simulink model "model2x2PulsedCA1ECMay1_2005"  (Simulink 7.1)
settings: Solver=ode45  StartTime=0.0  StopTime=100  RelTol=1e-3
settings Model: Creator=Terri Murray  LastModifiedBy=Terri Murray
settings DataIOCC: LimitDataPoints=off
settings OptimizationCC: InlineInvariantSignals=on
settings DebuggingCC: SaveWithParameterizedLinksMsg=none  SignalResolutionControl=TryResolveAllWithWarning  MultiTaskDSMMsg=warning  MultiTaskCondExecSysMsg=none  StrictBusMsg=None
settings RTWCC: IncludeERTFirstTime=on
settings GRTTargetCC: TargetFcnLib=ansi_tfl_tmw.mat

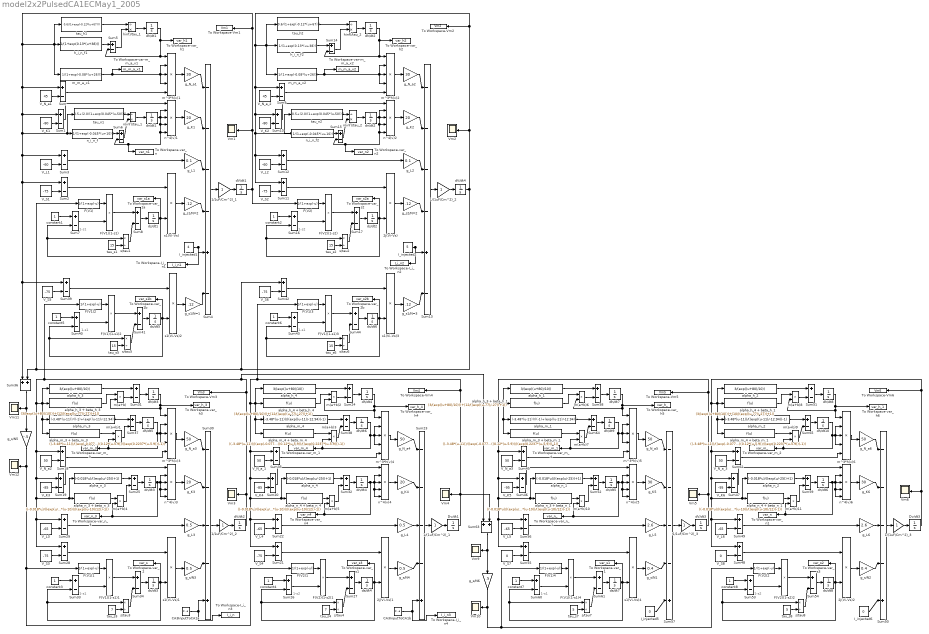
== system model2x2PulsedCA1ECMay1_2005 ==
  note: 1-s1
  note: 1-s2
  note: 1-s1
  note: 1-s2
  note: 1-s1
  note: 1-s1
  note: 1-s1
  note: 1-s2
  " 1/(1uF/Cm^2)_1" : Gain  ParameterDataType=sfix(16)  ParameterScaling=2^0  OutDataType=sfix(16)  OutScaling=2^0  SaturateOnIntegerOverflow=on  OutDataTypeStr=Inherit: Same as input  ParamDataTypeStr=Inherit: Same as input
  " 1/(1uF/Cm^2)_2" : Gain  ParameterDataType=sfix(16)  ParameterScaling=2^0  OutDataType=sfix(16)  OutScaling=2^0  SaturateOnIntegerOverflow=on  OutDataTypeStr=Inherit: Same as input  ParamDataTypeStr=Inherit: Same as input
  " 1/(1uF/Cm^2)_3" : Gain  ParameterDataType=sfix(16)  ParameterScaling=2^0  OutDataType=sfix(16)  OutScaling=2^0  SaturateOnIntegerOverflow=on  OutDataTypeStr=Inherit: Same as input  ParamDataTypeStr=Inherit: Same as input
  " 1/1uF/Cm^2)_1" : Gain  ParameterDataType=sfix(16)  ParameterScaling=2^0  OutDataType=sfix(16)  OutScaling=2^0  SaturateOnIntegerOverflow=on  OutDataTypeStr=Inherit: Same as input  ParamDataTypeStr=Inherit: Same as input
  " 1/1uF/Cm^2)_2" : Gain  ParameterDataType=sfix(16)  ParameterScaling=2^0  OutDataType=sfix(16)  OutScaling=2^0  SaturateOnIntegerOverflow=on  OutDataTypeStr=Inherit: Same as input  ParamDataTypeStr=Inherit: Same as input
  " 1/1uF/Cm^2)_3" : Gain  ParameterDataType=sfix(16)  ParameterScaling=2^0  OutDataType=sfix(16)  OutScaling=2^0  SaturateOnIntegerOverflow=on  OutDataTypeStr=Inherit: Same as input  ParamDataTypeStr=Inherit: Same as input
  2j(Vi-Vs) : Product  OutDataType=sfix(16)  OutScaling=2^0  RndMeth=Zero
  2j(Vi-Vs)1 : Product  OutDataType=sfix(16)  OutScaling=2^0  RndMeth=Zero
  2j(Vi-Vs)2 : Product  OutDataType=sfix(16)  OutScaling=2^0  RndMeth=Zero
  CA3InputToCA1a : DiscretePulseGenerator  PulseType=Time based  Amplitude=200  Period=.02  PulseWidth=2  PhaseDelay=.5
  CA3InputToCA1b : DiscretePulseGenerator  PulseType=Time based  Amplitude=200  Period=.02  PulseWidth=2
  Dv/dt1 : Integrator  InitialCondition=-67.6
  Dv/dt3 : Integrator  InitialCondition=-68
  F(V1){,1..4} (5 alike) : Fcn  Expr=1/(1+exp(-u))
  F(V1)(1-s1){,1..4} (5 alike) : Product  OutDataType=sfix(16)  OutScaling=2^0  RndMeth=Zero
  F(V2) : Fcn  Expr=1/(1+exp(-u))
  F(V2)(1-s2) : Product  OutDataType=sfix(16)  OutScaling=2^0  RndMeth=Zero
  F(V2)(1-s2)1 : Product  OutDataType=sfix(16)  OutScaling=2^0  RndMeth=Zero
  F(V2)(1-s2)2 : Product  OutDataType=sfix(16)  OutScaling=2^0  RndMeth=Zero
  F(V2)1 : Fcn  Expr=1/(1+exp(-u))
  F(V2)2 : Fcn  Expr=1/(1+exp(-u))
  I_injected1 : Constant  Value=4  OutDataType=sfix(16)  OutScaling=2^0
  I_injected2 : Constant  Value=5  OutDataType=sfix(16)  OutScaling=2^0
  I_injected5 : Constant  Value=0  OutDataType=sfix(16)  OutScaling=2^0
  I_injected6 : Constant  Value=0  OutDataType=sfix(16)  OutScaling=2^0
  Sum{,1..3,5..12,14..22,24..29,31..35,37..49,51..56,58..62,64..65} (58 alike) : Sum  Inputs=+-  OutDataType=sfix(16)  OutScaling=2^0  SaturateOnIntegerOverflow=on
  Sum13 : Sum  Inputs=-||-||-||-||+|||-  OutDataType=sfix(16)  OutScaling=2^0  SaturateOnIntegerOverflow=on
  Sum{23,30,50,57} (4 alike) : Sum  Inputs=-||-||-||-||+  OutDataType=sfix(16)  OutScaling=2^0  SaturateOnIntegerOverflow=on
  Sum36 : Sum  Orientation=down  OutDataType=sfix(16)  OutScaling=2^0  SaturateOnIntegerOverflow=on
  Sum4 : Sum  Inputs=-||-||-||-||+|||-  OutDataType=sfix(16)  OutScaling=2^0  SaturateOnIntegerOverflow=on
  Sum63 : Sum  Orientation=down  OutDataType=sfix(16)  OutScaling=2^0  SaturateOnIntegerOverflow=on
  To Workspace-I_i_n1 : ToWorkspace  VariableName=I_i_n1  SampleTime=-1  SaveFormat=Array
  To Workspace-I_i_n2 : ToWorkspace  VariableName=I_i_n2  SampleTime=-1  SaveFormat=Array
  To Workspace-I_i_n3 : ToWorkspace  VariableName=I_i_n  SampleTime=-1  SaveFormat=Array
  To Workspace-I_i_n4 : ToWorkspace  VariableName=I_i_n3  SampleTime=-1  SaveFormat=Array
  To Workspace-Vm1 : ToWorkspace  VariableName=Vm1  SampleTime=-1  SaveFormat=Array
  To Workspace-Vm2 : ToWorkspace  VariableName=Vm2  SampleTime=-1  SaveFormat=Array
  To Workspace-Vm3 : ToWorkspace  VariableName=Vm3  SampleTime=-1  SaveFormat=Array
  To Workspace-Vm4 : ToWorkspace  VariableName=Vm4  SampleTime=-1  SaveFormat=Array
  To Workspace-Vm5 : ToWorkspace  VariableName=Vm5  SampleTime=-1  SaveFormat=Array
  To Workspace-Vm6 : ToWorkspace  VariableName=Vm6  SampleTime=-1  SaveFormat=Array
  To Workspace-var-m_m_a_x1 : ToWorkspace  VariableName=m_m_a_x1  SampleTime=-1  SaveFormat=Array
  To Workspace-var-m_m_a_x2 : ToWorkspace  VariableName=m_m_a_x2  SampleTime=-1  SaveFormat=Array
  To Workspace-var_1 : ToWorkspace  VariableName=var_s1  SampleTime=-1  SaveFormat=Array
  To Workspace-var_1a : ToWorkspace  VariableName=var_s1a  SampleTime=-1  SaveFormat=Array
  To Workspace-var_1b : ToWorkspace  VariableName=var_s1b  SampleTime=-1  SaveFormat=Array
  To Workspace-var_2 : ToWorkspace  VariableName=var_s  SampleTime=-1  SaveFormat=Array
  To Workspace-var_2b : ToWorkspace  VariableName=var_s2b  SampleTime=-1  SaveFormat=Array
  To Workspace-var_h1 : ToWorkspace  VariableName=var_h1  SampleTime=-1  SaveFormat=Array
  To Workspace-var_h2 : ToWorkspace  VariableName=var_h2  SampleTime=-1  SaveFormat=Array
  To Workspace-var_h3 : ToWorkspace  VariableName=var_h_3  SampleTime=-1  SaveFormat=Array
  To Workspace-var_h4 : ToWorkspace  VariableName=var_h_4  SampleTime=-1  SaveFormat=Array
  To Workspace-var_h5 : ToWorkspace  VariableName=var_h_  SampleTime=-1  SaveFormat=Array
  To Workspace-var_h6 : ToWorkspace  VariableName=var_h_1  SampleTime=-1  SaveFormat=Array
  To Workspace-var_m_1 : ToWorkspace  VariableName=var_m_4  SampleTime=-1  SaveFormat=Array
  To Workspace-var_m_2 : ToWorkspace  VariableName=var_m_  SampleTime=-1  SaveFormat=Array
  To Workspace-var_m_3 : ToWorkspace  VariableName=var_m_3  SampleTime=-1  SaveFormat=Array
  To Workspace-var_m_4 : ToWorkspace  VariableName=var_m_1  SampleTime=-1  SaveFormat=Array
  To Workspace-var_n : ToWorkspace  VariableName=var_n1  SampleTime=-1  SaveFormat=Array
  To Workspace-var_n1 : ToWorkspace  VariableName=var_n  SampleTime=-1  SaveFormat=Array
  To Workspace-var_n2 : ToWorkspace  VariableName=var_n2  SampleTime=-1  SaveFormat=Array
  To Workspace-var_n4 : ToWorkspace  VariableName=var_n4  SampleTime=-1  SaveFormat=Array
  To Workspace-var_n_1 : ToWorkspace  VariableName=var_n_  SampleTime=-1  SaveFormat=Array
  To Workspace-var_n_3 : ToWorkspace  VariableName=var_n_3  SampleTime=-1  SaveFormat=Array
  To Workspace-var_s1 : ToWorkspace  VariableName=var_s3  SampleTime=-1  SaveFormat=Array
  To Workspace-var_s2 : ToWorkspace  VariableName=var_s2a  SampleTime=-1  SaveFormat=Array
  To Workspace-var_s3 : ToWorkspace  VariableName=var_s2  SampleTime=-1  SaveFormat=Array
  V_K1 : Constant  Value=-80  OutDataType=sfix(16)  OutScaling=2^0
  V_K2 : Constant  Value=-80  OutDataType=sfix(16)  OutScaling=2^0
  V_K3 : Constant  Value=-85  OutDataType=sfix(16)  OutScaling=2^0
  V_K4 : Constant  Value=-85  OutDataType=sfix(16)  OutScaling=2^0
  V_K5 : Constant  Value=-95  OutDataType=sfix(16)  OutScaling=2^0
  V_K6 : Constant  Value=-95  OutDataType=sfix(16)  OutScaling=2^0
  V_L1 : Constant  Value=-60  OutDataType=sfix(16)  OutScaling=2^0
  V_L2 : Constant  Value=-60  OutDataType=sfix(16)  OutScaling=2^0
  V_L{3..6} (4 alike) : Constant  Value=-65  OutDataType=sfix(16)  OutScaling=2^0
  V_N_a1 : Constant  Value=45  OutDataType=sfix(16)  OutScaling=2^0
  V_N_a2 : Constant  Value=50  OutDataType=sfix(16)  OutScaling=2^0
  V_N_a3 : Constant  Value=50  OutDataType=sfix(16)  OutScaling=2^0
  V_N_a_1 : Constant  Value=50  OutDataType=sfix(16)  OutScaling=2^0
  V_N_a_2 : Constant  Value=45  OutDataType=sfix(16)  OutScaling=2^0
  V_N_a_3 : Constant  Value=50  OutDataType=sfix(16)  OutScaling=2^0
  V_S{1..6} (6 alike) : Constant  Value=-75  OutDataType=sfix(16)  OutScaling=2^0
  V_S7 : Constant  Value=0  OutDataType=sfix(16)  OutScaling=2^0
  V_S8 : Constant  Value=0  OutDataType=sfix(16)  OutScaling=2^0
  Vm{1..6,9..12} (10 alike) : Scope
      Vm1 settings: TimeRange=100  YMin=-80  YMax=60  MaxDataPoints=100001
      Vm10 settings: TimeRange=2  YMin=-80  YMax=40  SaveName=ScopeData5  MaxDataPoints=100001
      Vm11 settings: TimeRange=2  YMin=-80  YMax=40  SaveName=ScopeData3  MaxDataPoints=100001
      Vm12 settings: TimeRange=2  YMin=-80  YMax=40  SaveName=ScopeData4  MaxDataPoints=100001
      Vm2 settings: TimeRange=100  YMin=-80  YMax=60  SaveName=ScopeData28  MaxDataPoints=100001
      Vm3 settings: TimeRange=100  YMin=-80  YMax=60  MaxDataPoints=100001
      Vm4 settings: TimeRange=100  YMin=-80  YMax=60  SaveName=ScopeData2  MaxDataPoints=100001
      Vm5 settings: TimeRange=100  YMin=-80  YMax=60  SaveName=ScopeData6  MaxDataPoints=100001
      Vm6 settings: TimeRange=100  YMin=-80  YMax=60  SaveName=ScopeData7  MaxDataPoints=100001
      Vm9 settings: TimeRange=2  YMin=-80  YMax=40  SaveName=ScopeData8  MaxDataPoints=100001
  alpha_h_{1..4} (4 alike) : Fcn  Expr=3/(exp((u+80)/10))
  alpha_h_3 + beta_h_1 : Fcn  Expr=(3/(exp((u+80)/10)))+(12/((exp((u-77)/-27))+1))
  alpha_h_3 + beta_h_3 : Fcn  Expr=(3/(exp((u+80)/10)))+(12/((exp((u-77)/-27))+1))
  alpha_h_4 + beta_h_1 : Fcn  Expr=(3/(exp((u+80)/10)))+(10/((exp((u-77)/-27))+1))
  alpha_h_4 + beta_h_4 : Fcn  Expr=(3/(exp((u+80)/10)))+(12/((exp((u-77)/-27))+1))
  alpha_m_1 : Fcn  Expr=(-3.48*(u-11))/((-1)+(exp((u-11)/-12.94)))
  alpha_m_2 : Fcn  Expr=(-3.48*(u-11))/((exp((u-11)/-12.94))-1)
  alpha_m_3 : Fcn  Expr=(-3.48*(u-11))/((-1)+(exp((u-11)/-12.94)))
  alpha_m_3 + beta_m_1 : Fcn  Expr=((-3.48*(u-11))/((exp(-0.0773*(u-11)))-1))+((0.12*(u-5.9))/((exp(0.2237*(u-5.9)))-1))
  alpha_m_3 + beta_m_3 : Fcn  Expr=((-3.48*(u-11))/((exp(-0.0773*(u-11)))-1))+((0.12*(u-5.9))/((exp(0.2237*(u-5.9)))-1))
  alpha_m_4 : Fcn  Expr=(-3.48*(u-11))/((exp((u-11)/-12.94))-1)
  alpha_m_4 + beta_m_1 : Fcn  Expr=((-3.48*(u-11))/((exp(-0.0773*(u-11)))-1))+((0.12*(u-5.9))/((exp(0.2237*(u-5.9)))-1))
  alpha_m_4 + beta_m_4 : Fcn  Expr=((-3.48*(u-11))/((exp(-0.0773*(u-11)))-1))+((0.12*(u-5.9))/((exp(0.2237*(u-5.9)))-1))
  alpha_n_{1..4} (4 alike) : Fcn  Expr=(-0.018*u)/((exp(u/-25))+1)
  alpha_n_3 + beta_n_1 : Fcn  Expr=((-0.018*u)/((exp(u/-25))-1))+((0.0036*(u-10))/((exp((u-10)/12))-1))
  alpha_n_3 + beta_n_3 : Fcn  Expr=((-0.018*u)/((exp(u/-25))-1))+((0.0036*(u-10))/((exp((u-10)/12))-1))
  alpha_n_4 + beta_n_1 : Fcn  Expr=((-0.018*u)/((exp(u/-25))-1))+((0.0036*(u-10))/((exp((u-10)/12))-1))
  alpha_n_4 + beta_n_4 : Fcn  Expr=((-0.018*u)/((exp(u/-25))-1))+((0.0036*(u-10))/((exp((u-10)/12))-1))
  constant{1..8} (8 alike) : Constant  OutDataType=sfix(16)  OutScaling=2^0
  dV/dt1 : Integrator  InitialCondition=-62
  dV/dt2 : Integrator  InitialCondition=-67.6
  dV/dt3 : Integrator  InitialCondition=-68
  dV/dt4 : Integrator  InitialCondition=-62
  dh/dt{1..4,7..8} (6 alike) : Integrator  InitialCondition=0.001
  dh/dt{5..6,9..10} (4 alike) : Integrator  InitialCondition=0.999
  dn/dt1 : Integrator
  dn/dt2 : Integrator
  dn/dt{3..6} (4 alike) : Integrator  InitialCondition=0.001
  ds/dt{1..8} (8 alike) : Integrator  InitialCondition=1
  g_K{1..4} (4 alike) : Gain  Gain=20  ParameterDataType=sfix(16)  ParameterScaling=2^0  OutDataType=sfix(16)  OutScaling=2^0  SaturateOnIntegerOverflow=on  OutDataTypeStr=Inherit: Same as input  ParamDataTypeStr=Inherit: Same as input
  g_K5 : Gain  Gain=30  ParameterDataType=sfix(16)  ParameterScaling=2^0  OutDataType=sfix(16)  OutScaling=2^0  SaturateOnIntegerOverflow=on  OutDataTypeStr=Inherit: Same as input  ParamDataTypeStr=Inherit: Same as input
  g_K6 : Gain  Gain=30  ParameterDataType=sfix(16)  ParameterScaling=2^0  OutDataType=sfix(16)  OutScaling=2^0  SaturateOnIntegerOverflow=on  OutDataTypeStr=Inherit: Same as input  ParamDataTypeStr=Inherit: Same as input
  g_L1 : Gain  Gain=0.1  ParameterDataType=sfix(16)  ParameterScaling=2^0  OutDataType=sfix(16)  OutScaling=2^0  SaturateOnIntegerOverflow=on  OutDataTypeStr=Inherit: Same as input  ParamDataTypeStr=Inherit: Same as input
  g_L2 : Gain  Gain=0.1  ParameterDataType=sfix(16)  ParameterScaling=2^0  OutDataType=sfix(16)  OutScaling=2^0  SaturateOnIntegerOverflow=on  OutDataTypeStr=Inherit: Same as input  ParamDataTypeStr=Inherit: Same as input
  g_L3 : Gain  Gain=0.5  ParameterDataType=sfix(16)  ParameterScaling=2^0  OutDataType=sfix(16)  OutScaling=2^0  SaturateOnIntegerOverflow=on  OutDataTypeStr=Inherit: Same as input  ParamDataTypeStr=Inherit: Same as input
  g_L4 : Gain  Gain=0.5  ParameterDataType=sfix(16)  ParameterScaling=2^0  OutDataType=sfix(16)  OutScaling=2^0  SaturateOnIntegerOverflow=on  OutDataTypeStr=Inherit: Same as input  ParamDataTypeStr=Inherit: Same as input
  g_L5 : Gain  Gain=2.6  ParameterDataType=sfix(16)  ParameterScaling=2^0  OutDataType=sfix(16)  OutScaling=2^0  SaturateOnIntegerOverflow=on  OutDataTypeStr=Inherit: Same as input  ParamDataTypeStr=Inherit: Same as input
  g_L6 : Gain  Gain=2.6  ParameterDataType=sfix(16)  ParameterScaling=2^0  OutDataType=sfix(16)  OutScaling=2^0  SaturateOnIntegerOverflow=on  OutDataTypeStr=Inherit: Same as input  ParamDataTypeStr=Inherit: Same as input
  g_N_a1 : Gain  Gain=30  ParameterDataType=sfix(16)  ParameterScaling=2^0  OutDataType=sfix(16)  OutScaling=2^0  SaturateOnIntegerOverflow=on  OutDataTypeStr=Inherit: Same as input  ParamDataTypeStr=Inherit: Same as input
  g_N_a2 : Gain  Gain=30  ParameterDataType=sfix(16)  ParameterScaling=2^0  OutDataType=sfix(16)  OutScaling=2^0  SaturateOnIntegerOverflow=on  OutDataTypeStr=Inherit: Same as input  ParamDataTypeStr=Inherit: Same as input
  g_N_a{3..6} (4 alike) : Gain  Gain=50  ParameterDataType=sfix(16)  ParameterScaling=2^0  OutDataType=sfix(16)  OutScaling=2^0  SaturateOnIntegerOverflow=on  OutDataTypeStr=Inherit: Same as input  ParamDataTypeStr=Inherit: Same as input
  g_s/N1 : Gain  Gain=0.4  ParameterDataType=sfix(16)  ParameterScaling=2^0  OutDataType=sfix(16)  OutScaling=2^0  SaturateOnIntegerOverflow=on  OutDataTypeStr=Inherit: Same as input  ParamDataTypeStr=Inherit: Same as input
  g_s/N2 : Gain  Gain=0.4  ParameterDataType=sfix(16)  ParameterScaling=2^0  OutDataType=sfix(16)  OutScaling=2^0  SaturateOnIntegerOverflow=on  OutDataTypeStr=Inherit: Same as input  ParamDataTypeStr=Inherit: Same as input
  g_s/N3 : Gain  Gain=0.5  ParameterDataType=sfix(16)  ParameterScaling=2^0  OutDataType=sfix(16)  OutScaling=2^0  SaturateOnIntegerOverflow=on  OutDataTypeStr=Inherit: Same as input  ParamDataTypeStr=Inherit: Same as input
  g_s/N4 : Gain  Gain=0.5  ParameterDataType=sfix(16)  ParameterScaling=2^0  OutDataType=sfix(16)  OutScaling=2^0  SaturateOnIntegerOverflow=on  OutDataTypeStr=Inherit: Same as input  ParamDataTypeStr=Inherit: Same as input
  g_s/N5 : Gain  Orientation=down  Gain=-.5  ParameterDataType=sfix(16)  ParameterScaling=2^0  OutDataType=sfix(16)  OutScaling=2^0  SaturateOnIntegerOverflow=on  OutDataTypeStr=Inherit: Same as input  ParamDataTypeStr=Inherit: Same as input
  g_s/N6 : Gain  Orientation=down  Gain=.5  ParameterDataType=sfix(16)  ParameterScaling=2^0  OutDataType=sfix(16)  OutScaling=2^0  SaturateOnIntegerOverflow=on  OutDataTypeStr=Inherit: Same as input  ParamDataTypeStr=Inherit: Same as input
  g_s1/N=1 : Gain  Gain=.12  ParameterDataType=sfix(16)  ParameterScaling=2^0  OutDataType=sfix(16)  OutScaling=2^0  SaturateOnIntegerOverflow=on  OutDataTypeStr=Inherit: Same as input  ParamDataTypeStr=Inherit: Same as input
  g_s1/N=2 : Gain  Gain=.12  ParameterDataType=sfix(16)  ParameterScaling=2^0  OutDataType=sfix(16)  OutScaling=2^0  SaturateOnIntegerOverflow=on  OutDataTypeStr=Inherit: Same as input  ParamDataTypeStr=Inherit: Same as input
  g_s1/N=3 : Gain  Gain=.12  ParameterDataType=sfix(16)  ParameterScaling=2^0  OutDataType=sfix(16)  OutScaling=2^0  SaturateOnIntegerOverflow=on  OutDataTypeStr=Inherit: Same as input  ParamDataTypeStr=Inherit: Same as input
  g_s2/N=2 : Gain  Gain=.12  ParameterDataType=sfix(16)  ParameterScaling=2^0  OutDataType=sfix(16)  OutScaling=2^0  SaturateOnIntegerOverflow=on  OutDataTypeStr=Inherit: Same as input  ParamDataTypeStr=Inherit: Same as input
  h_i_n_f1 : Fcn  Expr=1/(1+exp(0.13*(u+38)))
  h_i_n_f2 : Fcn  Expr=1/(1+exp(0.13*(u+38)))
  hinf)/tau_1 : Product  Inputs=/*  OutDataType=sfix(16)  OutScaling=2^-10
  hinf)/tau_2 : Product  Inputs=/*  OutDataType=sfix(16)  OutScaling=2^-10
  m(a+b){,1..11} (12 alike) : Product  OutDataType=sfix(16)  OutScaling=2^0  RndMeth=Zero
  m^3*h(v){1..6} (6 alike) : Product  Inputs=5  OutDataType=sfix(16)  OutScaling=2^0  RndMeth=Zero
  m_m_a_x1 : Fcn  Expr=1/(1+exp(-0.08*(u+26)))
  m_m_a_x2 : Fcn  Expr=1/(1+exp(-0.08*(u+26)))
  n(inf)/tau_1 : Product  Inputs=/*  OutDataType=sfix(16)  OutScaling=2^-10
  n(inf)/tau_2 : Product  Inputs=/*  OutDataType=sfix(16)  OutScaling=2^-10
  n^4(v){1..6} (6 alike) : Product  Inputs=5  OutDataType=sfix(16)  OutScaling=2^0  RndMeth=Zero
  n_i_n_f : Fcn  Expr=1/(1+exp(-0.045*(u+10)))
  n_i_n_f2 : Fcn  Expr=1/(1+exp(-0.045*(u+10)))
  s/tau{1..8} (8 alike) : Product  Inputs=*/  OutDataType=sfix(16)  OutScaling=2^-10
  s1(Vi-Vs){,1..4} (5 alike) : Product  OutDataType=sfix(16)  OutScaling=2^0  RndMeth=Zero
  tau_h1 : Fcn  Expr=0.6/(1+exp(-0.12*(u+67)))
  tau_h2 : Fcn  Expr=0.6/(1+exp(-0.12*(u+67)))
  tau_n1 : Fcn  Expr=0.5+(2.0/(1+exp(0.045*(u-50))))
  tau_n2 : Fcn  Expr=0.5+(2.0/(1+exp(0.045*(u-50))))
  tau_s{1..2,5..6} (4 alike) : Constant  Value=15  OutDataType=sfix(16)  OutScaling=2^0
  tau_s3 : Constant  Value=7  OutDataType=sfix(16)  OutScaling=2^0
  tau_s4 : Constant  Value=7  OutDataType=sfix(16)  OutScaling=2^0
  tau_s7 : Constant  Value=5  OutDataType=sfix(16)  OutScaling=2^0
  tau_s8 : Constant  Value=5  OutDataType=sfix(16)  OutScaling=2^0
  wires:
  V_N_a1/1 -> Sum/2
  V_K1/1 -> Sum1/2
  V_L1/1 -> Sum3/2
  Sum4/1 -> " 1/1uF/Cm^2)_1"/1
  V_S1/1 -> Sum2/2
  " 1/1uF/Cm^2)_1"/1 -> dV/dt1/1
  I_injected1/1 -> To Workspace-I_i_n1/1, Sum4/5
  g_N_a1/1 -> Sum4/1
  g_K1/1 -> Sum4/2
  g_L1/1 -> Sum4/3
  g_s1/N=2/1 -> Sum4/4
  Sum3/1 -> g_L1/1
  Sum1/1 -> n^4(v)1/1
  m^3*h(v)1/1 -> g_N_a1/1
  tau_h1/1 -> hinf)/tau_1/1
  Sum5/1 -> hinf)/tau_1/2
  hinf)/tau_1/1 -> dh/dt1/1
  dh/dt1/1 -> To Workspace-var_h1/1, Sum5/2, m^3*h(v)1/1
  n_i_n_f/1 -> Sum6/1
  tau_n1/1 -> n(inf)/tau_1/1
  Sum6/1 -> n(inf)/tau_1/2
  n(inf)/tau_1/1 -> dn/dt1/1
  dn/dt1/1 -> n^4(v)1/3, n^4(v)1/4, Sum6/2, To Workspace-var_n/1, n^4(v)1/5, n^4(v)1/2
  n^4(v)1/1 -> g_K1/1
  s1(Vi-Vs)/1 -> g_s1/N=2/1
  Sum2/1 -> s1(Vi-Vs)/1
  ds/dt1/1 -> To Workspace-var_1a/1, s1(Vi-Vs)/2, Sum7/2, s/tau1/1
  constant1/1 -> Sum7/1
  tau_s1/1 -> s/tau1/2
  s/tau1/1 -> Sum8/2
  Sum8/1 -> ds/dt1/1
  dV/dt1/1 -> Vm1/1, To Workspace-Vm1/1, Sum1/1, Sum3/1, Sum2/1, Sum36/1, Sum39/1, n_i_n_f/1, tau_n1/1, Sum/1, h_i_n_f1/1, tau_h1/1, m_m_a_x1/1, F(V2)/1
  h_i_n_f1/1 -> Sum5/1
  Sum/1 -> m^3*h(v)1/5
  m_m_a_x1/1 -> To Workspace-var-m_m_a_x1/1, m^3*h(v)1/2, m^3*h(v)1/4, m^3*h(v)1/3
  F(V1)(1-s1)/1 -> Sum8/1
  Sum7/1 -> F(V1)(1-s1)/2
  F(V1)/1 -> F(V1)(1-s1)/1
  V_N_a_2/1 -> Sum9/2
  V_K2/1 -> Sum10/2
  V_L2/1 -> Sum12/2
  V_S2/1 -> Sum11/2
  " 1/(1uF/Cm^2)_2"/1 -> dV/dt4/1
  I_injected2/1 -> Sum13/5, To Workspace-I_i_n2/1
  g_N_a2/1 -> Sum13/1
  g_K2/1 -> Sum13/2
  g_L2/1 -> Sum13/3
  g_s2/N=2/1 -> Sum13/4
  Sum12/1 -> g_L2/1
  Sum10/1 -> n^4(v)2/1
  m^3*h(v)2/1 -> g_N_a2/1
  tau_h2/1 -> hinf)/tau_2/1
  Sum14/1 -> hinf)/tau_2/2
  hinf)/tau_2/1 -> dh/dt2/1
  dh/dt2/1 -> m^3*h(v)2/1, Sum14/2, To Workspace-var_h2/1
  n_i_n_f2/1 -> Sum15/1
  tau_n2/1 -> n(inf)/tau_2/1
  Sum15/1 -> n(inf)/tau_2/2
  n(inf)/tau_2/1 -> dn/dt2/1
  dn/dt2/1 -> n^4(v)2/3, n^4(v)2/4, Sum15/2, To Workspace-var_n2/1, n^4(v)2/5, n^4(v)2/2
  n^4(v)2/1 -> g_K2/1
  2j(Vi-Vs)/1 -> g_s2/N=2/1
  Sum11/1 -> 2j(Vi-Vs)/1
  ds/dt2/1 -> To Workspace-var_s2/1, 2j(Vi-Vs)/2, Sum16/2, s/tau2/1
  constant2/1 -> Sum16/1
  tau_s2/1 -> s/tau2/2
  s/tau2/1 -> Sum17/2
  Sum17/1 -> ds/dt2/1
  dV/dt4/1 -> Vm2/1, To Workspace-Vm2/1, Sum10/1, Sum12/1, Sum11/1, n_i_n_f2/1, tau_n2/1, Sum9/1, h_i_n_f2/1, tau_h2/1, m_m_a_x2/1, Sum42/1, Sum36/2, F(V1)/1
  h_i_n_f2/1 -> Sum14/1
  Sum9/1 -> m^3*h(v)2/5
  m_m_a_x2/1 -> m^3*h(v)2/3, m^3*h(v)2/2, m^3*h(v)2/4, To Workspace-var-m_m_a_x2/1
  F(V2)(1-s2)/1 -> Sum17/1
  Sum16/1 -> F(V2)(1-s2)/2
  F(V2)/1 -> F(V2)(1-s2)/1
  V_N_a2/1 -> Sum18/2
  V_K3/1 -> Sum19/2
  V_L3/1 -> Sum29/2
  Sum30/1 -> " 1/1uF/Cm^2)_2"/1
  V_S3/1 -> Sum28/2
  " 1/1uF/Cm^2)_2"/1 -> dV/dt2/1
  CA3InputToCA1a/1 -> Sum30/5, To Workspace-I_i_n3/1
  g_N_a3/1 -> Sum30/1
  g_K3/1 -> Sum30/2
  g_L3/1 -> Sum30/3
  g_s/N3/1 -> Sum30/4
  Sum29/1 -> g_L3/1
  Sum19/1 -> n^4(v)3/1
  m^3*h(v)3/1 -> g_N_a3/1
  dh/dt3/1 -> To Workspace-var_h3/1, m^3*h(v)3/1, m(a+b)/2
  dn/dt3/1 -> n^4(v)3/3, n^4(v)3/4, n^4(v)3/5, n^4(v)3/2, m(a+b)4/2, To Workspace-var_n_3/1
  n^4(v)3/1 -> g_K3/1
  s1(Vi-Vs)1/1 -> g_s/N3/1
  Sum28/1 -> s1(Vi-Vs)1/1
  ds/dt3/1 -> To Workspace-var_2/1, s1(Vi-Vs)1/2, Sum33/2, s/tau3/1
  constant3/1 -> Sum33/1
  tau_s3/1 -> s/tau3/2
  s/tau3/1 -> Sum34/2
  Sum34/1 -> ds/dt3/1
  dV/dt2/1 -> Vm3/1, To Workspace-Vm3/1, Sum19/1, Sum29/1, Sum28/1, alpha_n_3 + beta_n_3/1, alpha_n_3/1, Sum18/1, alpha_h_3 + beta_h_3/1, alpha_h_3/1, alpha_m_3 + beta_m_3/1, alpha_m_3/1, F(V1)2/1, Sum63/1
  Sum18/1 -> m^3*h(v)3/5
  F(V1)(1-s1)1/1 -> Sum34/1
  Sum33/1 -> F(V1)(1-s1)1/2
  F(V1)1/1 -> F(V1)(1-s1)1/1
  V_N_a_1/1 -> Sum35/2
  V_K4/1 -> Sum20/2
  V_L4/1 -> Sum22/2
  Sum23/1 -> " 1/(1uF/Cm^2)_1"/1
  V_S4/1 -> Sum21/2
  " 1/(1uF/Cm^2)_1"/1 -> Dv/dt1/1
  CA3InputToCA1b/1 -> Sum23/5, To Workspace-I_i_n4/1
  g_N_a4/1 -> Sum23/1
  g_K4/1 -> Sum23/2
  g_L4/1 -> Sum23/3
  g_s/N4/1 -> Sum23/4
  Sum22/1 -> g_L4/1
  Sum20/1 -> n^4(v)4/1
  m^3*h(v)4/1 -> g_N_a4/1
  dn/dt4/1 -> n^4(v)4/3, n^4(v)4/4, n^4(v)4/5, n^4(v)4/2, To Workspace-var_n4/1, m(a+b)5/2
  n^4(v)4/1 -> g_K4/1
  2j(Vi-Vs)1/1 -> g_s/N4/1
  Sum21/1 -> 2j(Vi-Vs)1/1
  ds/dt4/1 -> To Workspace-var_s1/1, 2j(Vi-Vs)1/2, Sum26/2, s/tau4/1
  constant4/1 -> Sum26/1
  tau_s4/1 -> s/tau4/2
  s/tau4/1 -> Sum27/2
  Sum27/1 -> ds/dt4/1
  Dv/dt1/1 -> Vm4/1, To Workspace-Vm4/1, Sum20/1, Sum22/1, Sum21/1, alpha_n_4 + beta_n_4/1, alpha_n_4/1, Sum35/1, alpha_h_4 + beta_h_4/1, alpha_h_4/1, alpha_m_4/1, alpha_m_4 + beta_m_4/1, F(V1)3/1, Sum63/2
  Sum35/1 -> m^3*h(v)4/5
  F(V2)(1-s2)1/1 -> Sum27/1
  Sum26/1 -> F(V2)(1-s2)1/2
  F(V2)1/1 -> F(V2)(1-s2)1/1
  g_s/N5/1 -> Vm12/1, F(V1)1/1, F(V2)1/1
  Sum36/1 -> g_s/N5/1, Vm11/1
  alpha_h_3/1 -> Sum31/1
  m(a+b)/1 -> Sum31/2
  Sum31/1 -> dh/dt3/1
  alpha_h_3 + beta_h_3/1 -> m(a+b)/1
  alpha_m_3 + beta_m_3/1 -> m(a+b)1/1
  m(a+b)1/1 -> Sum37/2
  alpha_m_3/1 -> Sum37/1
  Sum37/1 -> dh/dt5/1
  dh/dt5/1 -> m^3*h(v)3/3, m^3*h(v)3/2, m^3*h(v)3/4, m(a+b)1/2, To Workspace-var_m_3/1
  m(a+b)2/1 -> Sum24/2
  Sum24/1 -> dh/dt4/1
  dh/dt4/1 -> To Workspace-var_h4/1, m^3*h(v)4/1, m(a+b)2/2
  Sum38/1 -> dh/dt6/1
  m(a+b)3/1 -> Sum38/2
  dh/dt6/1 -> m^3*h(v)4/3, m^3*h(v)4/2, m^3*h(v)4/4, m(a+b)3/2, To Workspace-var_m_1/1
  alpha_h_4/1 -> Sum24/1
  alpha_h_4 + beta_h_4/1 -> m(a+b)2/1
  alpha_m_4/1 -> Sum38/1
  alpha_m_4 + beta_m_4/1 -> m(a+b)3/1
  Sum25/1 -> dn/dt3/1
  alpha_n_3/1 -> Sum25/1
  alpha_n_3 + beta_n_3/1 -> m(a+b)4/1
  m(a+b)4/1 -> Sum25/2
  Sum32/1 -> dn/dt4/1
  alpha_n_4/1 -> Sum32/1
  alpha_n_4 + beta_n_4/1 -> m(a+b)5/1
  m(a+b)5/1 -> Sum32/2
  V_S5/1 -> Sum39/2
  s1(Vi-Vs)2/1 -> g_s1/N=1/1
  Sum39/1 -> s1(Vi-Vs)2/1
  ds/dt5/1 -> s1(Vi-Vs)2/2, Sum40/2, s/tau5/1, To Workspace-var_1b/1
  constant5/1 -> Sum40/1
  tau_s5/1 -> s/tau5/2
  s/tau5/1 -> Sum41/2
  Sum41/1 -> ds/dt5/1
  F(V1)(1-s1)2/1 -> Sum41/1
  Sum40/1 -> F(V1)(1-s1)2/2
  F(V1)2/1 -> F(V1)(1-s1)2/1
  V_S6/1 -> Sum42/2
  s1(Vi-Vs)3/1 -> g_s1/N=3/1
  Sum42/1 -> s1(Vi-Vs)3/1
  ds/dt6/1 -> To Workspace-var_2b/1, s1(Vi-Vs)3/2, Sum43/2, s/tau6/1
  constant6/1 -> Sum43/1
  tau_s6/1 -> s/tau6/2
  s/tau6/1 -> Sum44/2
  Sum44/1 -> ds/dt6/1
  F(V1)(1-s1)3/1 -> Sum44/1
  Sum43/1 -> F(V1)(1-s1)3/2
  F(V1)3/1 -> F(V1)(1-s1)3/1
  Sum13/1 -> " 1/(1uF/Cm^2)_2"/1
  g_s1/N=1/1 -> Sum4/6
  g_s1/N=3/1 -> Sum13/6
  V_N_a3/1 -> Sum45/2
  V_K5/1 -> Sum46/2
  V_L5/1 -> Sum56/2
  Sum57/1 -> " 1/1uF/Cm^2)_3"/1
  V_S7/1 -> Sum55/2
  " 1/1uF/Cm^2)_3"/1 -> dV/dt3/1
  g_N_a5/1 -> Sum57/1
  g_K5/1 -> Sum57/2
  g_L5/1 -> Sum57/3
  g_s/N1/1 -> Sum57/4
  Sum56/1 -> g_L5/1
  Sum46/1 -> n^4(v)5/1
  m^3*h(v)5/1 -> g_N_a5/1
  dh/dt7/1 -> To Workspace-var_h5/1, m^3*h(v)5/1, m(a+b)6/2
  dn/dt5/1 -> n^4(v)5/3, n^4(v)5/4, n^4(v)5/5, n^4(v)5/2, m(a+b)10/2, To Workspace-var_n_1/1
  n^4(v)5/1 -> g_K5/1
  s1(Vi-Vs)4/1 -> g_s/N1/1
  Sum55/1 -> s1(Vi-Vs)4/1
  ds/dt7/1 -> To Workspace-var_1/1, s1(Vi-Vs)4/2, Sum60/2, s/tau7/1
  constant7/1 -> Sum60/1
  tau_s7/1 -> s/tau7/2
  s/tau7/1 -> Sum61/2
  Sum61/1 -> ds/dt7/1
  dV/dt3/1 -> Vm5/1, To Workspace-Vm5/1, Sum46/1, Sum56/1, Sum55/1, alpha_n_3 + beta_n_1/1, alpha_n_1/1, Sum45/1, alpha_h_3 + beta_h_1/1, alpha_h_1/1, alpha_m_3 + beta_m_1/1, alpha_m_1/1
  Sum45/1 -> m^3*h(v)5/5
  F(V1)(1-s1)4/1 -> Sum61/1
  Sum60/1 -> F(V1)(1-s1)4/2
  F(V1)4/1 -> F(V1)(1-s1)4/1
  V_N_a_3/1 -> Sum62/2
  V_K6/1 -> Sum47/2
  V_L6/1 -> Sum49/2
  Sum50/1 -> " 1/(1uF/Cm^2)_3"/1
  V_S8/1 -> Sum48/2
  " 1/(1uF/Cm^2)_3"/1 -> Dv/dt3/1
  g_N_a6/1 -> Sum50/1
  g_K6/1 -> Sum50/2
  g_L6/1 -> Sum50/3
  g_s/N2/1 -> Sum50/4
  Sum49/1 -> g_L6/1
  Sum47/1 -> n^4(v)6/1
  m^3*h(v)6/1 -> g_N_a6/1
  dn/dt6/1 -> n^4(v)6/3, n^4(v)6/4, n^4(v)6/5, n^4(v)6/2, To Workspace-var_n1/1, m(a+b)11/2
  n^4(v)6/1 -> g_K6/1
  2j(Vi-Vs)2/1 -> g_s/N2/1
  Sum48/1 -> 2j(Vi-Vs)2/1
  ds/dt8/1 -> To Workspace-var_s3/1, 2j(Vi-Vs)2/2, Sum53/2, s/tau8/1
  constant8/1 -> Sum53/1
  tau_s8/1 -> s/tau8/2
  s/tau8/1 -> Sum54/2
  Sum54/1 -> ds/dt8/1
  Dv/dt3/1 -> To Workspace-Vm6/1, Sum47/1, Sum49/1, Sum48/1, alpha_n_4 + beta_n_1/1, alpha_n_2/1, Sum62/1, alpha_h_4 + beta_h_1/1, alpha_h_2/1, alpha_m_2/1, alpha_m_4 + beta_m_1/1, Vm6/1
  Sum62/1 -> m^3*h(v)6/5
  F(V2)(1-s2)2/1 -> Sum54/1
  Sum53/1 -> F(V2)(1-s2)2/2
  F(V2)2/1 -> F(V2)(1-s2)2/1
  g_s/N6/1 -> Vm10/1, F(V1)4/1, F(V2)2/1
  Sum63/1 -> g_s/N6/1, Vm9/1
  alpha_h_1/1 -> Sum58/1
  m(a+b)6/1 -> Sum58/2
  Sum58/1 -> dh/dt7/1
  alpha_h_3 + beta_h_1/1 -> m(a+b)6/1
  alpha_m_3 + beta_m_1/1 -> m(a+b)7/1
  m(a+b)7/1 -> Sum64/2
  alpha_m_1/1 -> Sum64/1
  Sum64/1 -> dh/dt9/1
  dh/dt9/1 -> m^3*h(v)5/3, m^3*h(v)5/2, m^3*h(v)5/4, m(a+b)7/2, To Workspace-var_m_4/1
  m(a+b)8/1 -> Sum51/2
  Sum51/1 -> dh/dt8/1
  dh/dt8/1 -> To Workspace-var_h6/1, m^3*h(v)6/1, m(a+b)8/2
  Sum65/1 -> dh/dt10/1
  m(a+b)9/1 -> Sum65/2
  dh/dt10/1 -> m^3*h(v)6/3, m^3*h(v)6/2, m^3*h(v)6/4, m(a+b)9/2, To Workspace-var_m_2/1
  alpha_h_2/1 -> Sum51/1
  alpha_h_4 + beta_h_1/1 -> m(a+b)8/1
  alpha_m_2/1 -> Sum65/1
  alpha_m_4 + beta_m_1/1 -> m(a+b)9/1
  Sum52/1 -> dn/dt5/1
  alpha_n_1/1 -> Sum52/1
  alpha_n_3 + beta_n_1/1 -> m(a+b)10/1
  m(a+b)10/1 -> Sum52/2
  Sum59/1 -> dn/dt6/1
  alpha_n_2/1 -> Sum59/1
  alpha_n_4 + beta_n_1/1 -> m(a+b)11/1
  m(a+b)11/1 -> Sum59/2
  I_injected6/1 -> Sum50/5
  I_injected5/1 -> Sum57/5
